simulink model "HANcoder_E407_TTA_Group2"  (R2018b)
settings: Solver=FixedStepDiscrete  StartTime=0.0  StopTime=1  FixedStep=0.01  RelTol=1e-3
PreLoadFcn:
  | librarySetup
  | eval([bdroot,'_startup']) %Calling [modelName]_startup.m
values from neighbouring files (symbols this model uses):
  BackUp_Role = 4    [HANcoder_E407_TTA_Group2_startup.m]
  basic_cycle_duration_bc0 = TM_Reset_Board   + COMP_duration    (= 550)    [HANcoder_E407_TTA_Group2_startup.m]    (also in HANcoder_E407_TTA_Template_startup.m = 212)
  basic_cycle_duration_bc1 = TM_Reset_Var_bc1 + COMP_duration    (= 610)    [HANcoder_E407_TTA_Group2_startup.m]    (also in HANcoder_E407_TTA_Template_startup.m = 212)
  board1_online = Simulink.Parameter    [HANcoder_E407_TTA_Group2_startup.m]
  board2_online = Simulink.Parameter    [HANcoder_E407_TTA_Group2_startup.m]
  board3_online = Simulink.Parameter    [HANcoder_E407_TTA_Group2_startup.m]
  board4_online = Simulink.Parameter    [HANcoder_E407_TTA_Group2_startup.m]
  comm_delay_estimation1 = round(comm_delay_measured1*hardware_granularity/frequency_IRQ)    [HANcoder_E407_TTA_Group2_startup.m]    (also in HANcoder_E407_TTA_Template_startup.m)
  comm_delay_estimation2 = round(comm_delay_measured2*hardware_granularity/frequency_IRQ)    [HANcoder_E407_TTA_Group2_startup.m]    (also in HANcoder_E407_TTA_Template_startup.m)
  COMM_Period = 50    [HANcoder_E407_TTA_Group2_startup.m]    (also in HANcoder_E407_TTA_Template_startup.m = 40)
  COMM_Phase1 = Simulink.Parameter    [HANcoder_E407_TTA_Group2_startup.m]    (also in HANcoder_E407_TTA_Template_startup.m)
  COMM_Phase2 = Simulink.Parameter    [HANcoder_E407_TTA_Group2_startup.m]    (also in HANcoder_E407_TTA_Template_startup.m)
  COMM_Phase_init1 = Simulink.Parameter    [HANcoder_E407_TTA_Group2_startup.m]    (also in HANcoder_E407_TTA_Template_startup.m)
  COMM_Phase_init2 = Simulink.Parameter    [HANcoder_E407_TTA_Group2_startup.m]    (also in HANcoder_E407_TTA_Template_startup.m)
  COMP_duration = 20    [HANcoder_E407_TTA_Group2_startup.m]    (also in HANcoder_E407_TTA_Template_startup.m = 4)
  Controller1_Board = 1    [HANcoder_E407_TTA_Group2_startup.m]    (also in HANcoder_E407_TTA_Template_startup.m)
  Controller2_Board = 2    [HANcoder_E407_TTA_Group2_startup.m]    (also in HANcoder_E407_TTA_Template_startup.m)
  Controller3_Board = 3    [HANcoder_E407_TTA_Group2_startup.m]    (also in HANcoder_E407_TTA_Template_startup.m)
  Controller4_Board = 4    [HANcoder_E407_TTA_Group2_startup.m]
  delta_a_set = Simulink.Parameter    [HANcoder_E407_TTA_Group2_startup.m]
  delta_f_set = Simulink.Parameter    [HANcoder_E407_TTA_Group2_startup.m]
  delta_max = 1    [HANcoder_E407_TTA_Group2_startup.m]
  delta_min = -1    [HANcoder_E407_TTA_Group2_startup.m]
  delta_precision = 6    [HANcoder_E407_TTA_Group2_startup.m]
  e_width = 0.1    [HANcoder_E407_TTA_Group2_startup.m]
  ErrorLog_ID = 31    [HANcoder_E407_TTA_Group2_startup.m]
  frequency_IRQ = 100    [HANcoder_E407_TTA_Group2_startup.m]    (also in HANcoder_E407_TTA_Template_startup.m)
  HANtuneOverride = Simulink.Parameter    [HANcoder_E407_TTA_Group2_startup.m]    (also in HANcoder_E407_TTA_Template_startup.m)
  hardware_granularity = 1000000    [HANcoder_E407_TTA_Group2_startup.m]    (also in HANcoder_E407_TTA_Template_startup.m)
  I_a = 2.25    [HANcoder_E407_TTA_Group2_startup.m]
  I_f = 2.25    [HANcoder_E407_TTA_Group2_startup.m]
  idle_time_init = basic_cycle_duration_bc0 + basic_cycle_duration_bc1    (= 1160)    [HANcoder_E407_TTA_Group2_startup.m]    (also in HANcoder_E407_TTA_Template_startup.m = 424)
  Input_Gen_Board = 5    [HANcoder_E407_TTA_Group2_startup.m]
  LA_Clock_Gr = 1    [HANcoder_E407_TTA_Group2_startup.m]    (also in HANcoder_E407_TTA_Template_startup.m)
  LA_COMM_dly = 1    [HANcoder_E407_TTA_Group2_startup.m]    (also in HANcoder_E407_TTA_Template_startup.m)
  LA_COMM_Err = 1    [HANcoder_E407_TTA_Group2_startup.m]    (also in HANcoder_E407_TTA_Template_startup.m)
  LA_E_Desync = 1    [HANcoder_E407_TTA_Group2_startup.m]    (also in HANcoder_E407_TTA_Template_startup.m)
  LA_MEX_Flag = 1    [HANcoder_E407_TTA_Group2_startup.m]    (also in HANcoder_E407_TTA_Template_startup.m)
  LA_Task_Act = 1    [HANcoder_E407_TTA_Group2_startup.m]    (also in HANcoder_E407_TTA_Template_startup.m)
  m_v = 100.0    (= 100)    [HANcoder_E407_TTA_Group2_startup.m]
  Master_Role = 1    [HANcoder_E407_TTA_Group2_startup.m]    (also in HANcoder_E407_TTA_Template_startup.m)
  matrix_cycle_duration = basic_cycle_duration_bc0 + basic_cycle_duration_bc1    (= 1160)    [HANcoder_E407_TTA_Group2_startup.m]    (also in HANcoder_E407_TTA_Template_startup.m = 424)
  matrix_rows = 2    [HANcoder_E407_TTA_Group2_startup.m]    (also in HANcoder_E407_TTA_Template_startup.m)
  max_desync = 15    [HANcoder_E407_TTA_Group2_startup.m]    (also in HANcoder_E407_TTA_Template_startup.m)
  max_num_msgs_CAN1 = 2^Tx_bit_number-1    (= 7)    [HANcoder_E407_TTA_Group2_startup.m]    (also in HANcoder_E407_TTA_Template_startup.m)
  max_num_msgs_CAN2 = max_num_msgs_CAN1    (= 7)    [HANcoder_E407_TTA_Group2_startup.m]    (also in HANcoder_E407_TTA_Template_startup.m)
  min_desync = (-1)*max_desync    (= -15)    [HANcoder_E407_TTA_Group2_startup.m]    (also in HANcoder_E407_TTA_Template_startup.m)
  OutControl1_ID = 23    [HANcoder_E407_TTA_Group2_startup.m]    (also in HANcoder_E407_TTA_Template_startup.m)
  OutControl2_ID = 24    [HANcoder_E407_TTA_Group2_startup.m]    (also in HANcoder_E407_TTA_Template_startup.m)
  OutEmulator_ID = 25    [HANcoder_E407_TTA_Group2_startup.m]    (also in HANcoder_E407_TTA_Template_startup.m)
  R_al = 0.10    (= 0.1)    [HANcoder_E407_TTA_Group2_startup.m]
  R_ar = 0.10    (= 0.1)    [HANcoder_E407_TTA_Group2_startup.m]
  R_fl = 0.10    (= 0.1)    [HANcoder_E407_TTA_Group2_startup.m]
  R_fr = 0.10    (= 0.1)    [HANcoder_E407_TTA_Group2_startup.m]
  script_run = Simulink.Parameter    [HANcoder_E407_TTA_Group2_startup.m]    (also in HANcoder_E407_TTA_Template_startup.m)
  SensorValues_ID = 22    [HANcoder_E407_TTA_Group2_startup.m]    (also in HANcoder_E407_TTA_Template_startup.m)
  SetValues_ID = 21    [HANcoder_E407_TTA_Group2_startup.m]    (also in HANcoder_E407_TTA_Template_startup.m)
  Slave_Role = 3    [HANcoder_E407_TTA_Group2_startup.m]    (also in HANcoder_E407_TTA_Template_startup.m = 2)
  speed_k_d = Simulink.Parameter    [HANcoder_E407_TTA_Group2_startup.m]
  speed_k_i = Simulink.Parameter    [HANcoder_E407_TTA_Group2_startup.m]
  speed_k_p = Simulink.Parameter    [HANcoder_E407_TTA_Group2_startup.m]
  speed_max = 10    [HANcoder_E407_TTA_Group2_startup.m]
  speed_min = -10    [HANcoder_E407_TTA_Group2_startup.m]
  speed_precision = 3    [HANcoder_E407_TTA_Group2_startup.m]
  Sync_ID = 1    [HANcoder_E407_TTA_Group2_startup.m]    (also in HANcoder_E407_TTA_Template_startup.m)
  tau_max = 5    [HANcoder_E407_TTA_Group2_startup.m]
  tau_min = -5    [HANcoder_E407_TTA_Group2_startup.m]
  tau_range = abs(tau_max) + abs(tau_min)    [HANcoder_E407_TTA_Group2_startup.m]
  theta_max = (speed_max/R_fr)*matrix_cycle_duration*frequency_IRQ/hardware_granularity    (= 11.6)    [HANcoder_E407_TTA_Group2_startup.m]
  theta_min = (-1)*theta_max    (= -11.6)    [HANcoder_E407_TTA_Group2_startup.m]
  theta_precision = 7-(fix(log2(theta_max))+1)    [HANcoder_E407_TTA_Group2_startup.m]
  Tl_a = 0.6    [HANcoder_E407_TTA_Group2_startup.m]
  Tl_f = 0.6    [HANcoder_E407_TTA_Group2_startup.m]
  TM_bc0_1 = basic_cycle_start    (= 0)    [HANcoder_E407_TTA_Group2_startup.m]
  TM_bc0_10 = TM_bc0_9 + COMP_duration    (= 270)    [HANcoder_E407_TTA_Group2_startup.m]
  TM_bc0_11 = TM_bc0_10 + COMP_duration    (= 290)    [HANcoder_E407_TTA_Group2_startup.m]
  TM_bc0_12 = TM_bc0_11  + COMM_duration    (= 340)    [HANcoder_E407_TTA_Group2_startup.m]
  TM_bc0_13 = TM_bc0_12 + COMP_duration    (= 360)    [HANcoder_E407_TTA_Group2_startup.m]
  TM_bc0_14 = TM_bc0_13 + COMP_duration    (= 380)    [HANcoder_E407_TTA_Group2_startup.m]
  TM_bc0_15 = TM_bc0_14  + COMM_duration    (= 430)    [HANcoder_E407_TTA_Group2_startup.m]
  TM_bc0_16 = TM_bc0_15 + COMP_duration    (= 450)    [HANcoder_E407_TTA_Group2_startup.m]
  TM_bc0_17 = TM_bc0_16 + COMP_duration    (= 470)    [HANcoder_E407_TTA_Group2_startup.m]
  TM_bc0_18 = TM_bc0_17 + COMP_duration    (= 490)    [HANcoder_E407_TTA_Group2_startup.m]
  TM_bc0_2 = TM_bc0_1   + COMM_duration    (= 50)    [HANcoder_E407_TTA_Group2_startup.m]
  TM_bc0_3 = TM_bc0_2  + COMP_duration    (= 70)    [HANcoder_E407_TTA_Group2_startup.m]
  TM_bc0_3_2 = TM_bc0_3   + 2    (= 72)    [HANcoder_E407_TTA_Group2_startup.m]
  TM_bc0_4 = TM_bc0_3   + COMP_duration    (= 90)    [HANcoder_E407_TTA_Group2_startup.m]
  TM_bc0_4_2 = TM_bc0_4    + 2    (= 92)    [HANcoder_E407_TTA_Group2_startup.m]
  TM_bc0_5 = TM_bc0_4    + COMP_duration    (= 110)    [HANcoder_E407_TTA_Group2_startup.m]
  TM_bc0_6 = TM_bc0_5  + COMM_duration    (= 160)    [HANcoder_E407_TTA_Group2_startup.m]
  TM_bc0_7 = TM_bc0_6 + COMP_duration    (= 180)    [HANcoder_E407_TTA_Group2_startup.m]
  TM_bc0_8 = TM_bc0_7 + COMP_duration    (= 200)    [HANcoder_E407_TTA_Group2_startup.m]
  TM_bc0_9 = TM_bc0_8  + COMM_duration    (= 250)    [HANcoder_E407_TTA_Group2_startup.m]
  TM_bc0_9_2 = TM_bc0_9 + 2    (= 252)    [HANcoder_E407_TTA_Group2_startup.m]
  TM_bc1_18 = TM_Check_Output_Emulator + COMP_duration    (= 520)    [HANcoder_E407_TTA_Group2_startup.m]
  TM_bc1_19 = TM_bc1_18 + COMM_duration    (= 570)    [HANcoder_E407_TTA_Group2_startup.m]
  TM_bc1_19_2 = TM_bc1_19 + 2    (= 572)    [HANcoder_E407_TTA_Group2_startup.m]
  TM_Check_Output_Control1 = TM_COMM_Output_Control1 + COMP_duration    (= 340)    [HANcoder_E407_TTA_Group2_startup.m]
  TM_Check_Output_Control2 = TM_COMM_Output_Control2 + COMM_duration    (= 410)    [HANcoder_E407_TTA_Group2_startup.m]
  TM_Check_Output_Emulator = TM_COMM_Output_Emulator + COMM_duration    (= 500)    [HANcoder_E407_TTA_Group2_startup.m]
  TM_Check_Output_Emulator_2 = TM_Check_Output_Emulator + 2    (= 502)    [HANcoder_E407_TTA_Group2_startup.m]
  TM_Check_Sensor_Values = TM_COMM_Sensor_Values + COMM_duration    (= 210)    [HANcoder_E407_TTA_Group2_startup.m]
  TM_Check_Sensor_Values_2 = TM_Check_Sensor_Values + 2    (= 212)    [HANcoder_E407_TTA_Group2_startup.m]
  TM_Check_Set_Values = TM_COMM_Set_Values + COMM_duration    (= 140)    [HANcoder_E407_TTA_Group2_startup.m]
  TM_Check_Set_Values_2 = TM_Check_Set_Values + 2    (= 142)    [HANcoder_E407_TTA_Group2_startup.m]
  TM_COMM_Output_Control1 = TM_Velocity + COMM_duration    (= 320)    [HANcoder_E407_TTA_Group2_startup.m]
  TM_COMM_Output_Control2 = TM_Check_Output_Control1 + COMP_duration    (= 360)    [HANcoder_E407_TTA_Group2_startup.m]
  TM_COMM_Output_Emulator = TM_TMR + COMP_duration    (= 450)    [HANcoder_E407_TTA_Group2_startup.m]
  TM_COMM_Sensor_Values = TM_Check_Set_Values + COMP_duration    (= 160)    [HANcoder_E407_TTA_Group2_startup.m]
  TM_COMM_Set_Values = TM_bc0_3 + COMP_duration    (= 90)    [HANcoder_E407_TTA_Group2_startup.m]
  TM_COMM_Sync = basic_cycle_start    (= 0)    [HANcoder_E407_TTA_Group2_startup.m]    (also in HANcoder_E407_TTA_Template_startup.m)
  TM_Data_bc0 = TM_COMM_Sync    (= 0)    [HANcoder_E407_TTA_Group2_startup.m]    (also in HANcoder_E407_TTA_Template_startup.m)
  TM_Data_bc1 = TM_Data_bc0(1:4)    [HANcoder_E407_TTA_Group2_startup.m]    (also in HANcoder_E407_TTA_Template_startup.m)
  TM_Reset_Board = TM_Reset_Var   + COMP_duration    (= 530)    [HANcoder_E407_TTA_Group2_startup.m]    (also in HANcoder_E407_TTA_Template_startup.m = 208)
  TM_Reset_Var = TM_bc0_18  + COMP_duration    (= 510)    [HANcoder_E407_TTA_Group2_startup.m]    (also in HANcoder_E407_TTA_Template_startup.m = 204)
  TM_Reset_Var_bc1 = TM_bc1_19 + COMP_duration    (= 590)    [HANcoder_E407_TTA_Group2_startup.m]    (also in HANcoder_E407_TTA_Template_startup.m = 200)
  TM_Reset_Var_bc1_2 = TM_Reset_Var_bc1 + 2    (= 592)    [HANcoder_E407_TTA_Group2_startup.m]    (also in HANcoder_E407_TTA_Template_startup.m = 202)
  TM_Steer = TM_Check_Sensor_Values + COMP_duration    (= 230)    [HANcoder_E407_TTA_Group2_startup.m]
  TM_TMR = TM_Check_Output_Control2 + COMP_duration    (= 430)    [HANcoder_E407_TTA_Group2_startup.m]
  TM_TMR_2 = TM_TMR + 1    (= 431)    [HANcoder_E407_TTA_Group2_startup.m]
  ... (+19 more)
undefined symbols (not defined in the file or in its folder): A0, A1, A2, A3, A4, CON2, CON4, D10, D12, D13, D8, D9
libraries: hdlsllib x340, HANcoder_STM32_Target x28, simulink x5, simulink_extras x1
(part 21 of 36)

== system HANcoder_E407_TTA_Group2/HANcoder STM32 Target - E407-STM32 algorithm/TTA CAN System/TTA System/Matrix Cycle Manager/Controller Matrix Cycle/controller basic cycle 0/COMM Task - Vote4/Transmission subtasks/Check msg transmission CAN1 ==
  note: The TX buffers are updated one tick
      | before the message is sent
  note: A message should be sent during
      | this tick through CAN1
  note: In the next tick, a message will be
      | sent through CAN1
  Local Time : Inport
  Time Mark : Inport  Port=2
  Tx_ID : Inport  Port=3
  Value Domain Msg : Inport  Port=4
  Enable : EnablePort
  Constant : Constant  Value=COMM_Phase_init1
  Constant11 : Constant  Value=0
  Constant22 : Constant
  Constant24 : Constant  Value=COMM_Phase1
  Constant27 : Constant  Value=COMM_Phase1
  Constant8 : Constant  Value=0
  Equal4 : RelationalOperator  Operator===  OutDataTypeStr=boolean  RndMeth=Simplest
  Equal7 : RelationalOperator  Operator===  OutDataTypeStr=boolean  RndMeth=Simplest
  Minus : Sum  Inputs=++-
  Minus1 : Sum  Inputs=+-
  Minus2 : Sum
  Mod : Math  Operator=mod  SaturateOnIntegerOverflow=on
  Mod1 : Math  Operator=mod  SaturateOnIntegerOverflow=on
  TX buffer update CAN1 : Subsystem  Priority=20
  Send CAN1 : Outport  OutputWhenDisabled=reset  InitialOutput=0
  wires:
  Equal4/1 -> TX buffer update CAN1/Enable
  Constant22/1 -> Minus/2
  Local Time/1 -> Minus1/1, Minus/1
  Tx_ID/1 -> TX buffer update CAN1/1(Tx_ID)
  Mod1/1 -> Equal7/1
  Constant27/1 -> Mod1/2
  Minus/1 -> Mod/1
  Value Domain Msg/1 -> TX buffer update CAN1/2(Msg_Value_Data)
  Constant24/1 -> Mod/2
  Mod/1 -> Equal4/1
  Minus1/1 -> Mod1/1
  Constant11/1 -> Equal7/2
  Equal7/1 -> Send CAN1/1
  Constant8/1 -> Equal4/2
  Constant/1 -> Minus2/2
  Minus2/1 -> Minus1/2, Minus/3
  Time Mark/1 -> Minus2/1

== system HANcoder_E407_TTA_Group2/HANcoder STM32 Target - E407-STM32 algorithm/TTA CAN System/TTA System/Matrix Cycle Manager/Controller Matrix Cycle/controller basic cycle 0/COMM Task - Vote4/Transmission subtasks/Check msg transmission CAN2 ==
  note: In the next tick, a message will be
      | sent through CAN2
  note: A message should be sent during
      | this tick through CAN2
  note: The TX buffers are updated one tick
      | before the message is sent
  Local Time : Inport
  Time Mark : Inport  Port=2
  Tx_ID : Inport  Port=3
  Value Domain Msg : Inport  Port=4
  Enable : EnablePort
  Constant : Constant  Value=COMM_Phase_init2
  Constant11 : Constant  Value=0
  Constant22 : Constant
  Constant24 : Constant  Value=COMM_Phase2
  Constant27 : Constant  Value=COMM_Phase2
  Constant8 : Constant  Value=0
  Equal4 : RelationalOperator  Operator===  OutDataTypeStr=boolean  RndMeth=Simplest
  Equal7 : RelationalOperator  Operator===  OutDataTypeStr=boolean  RndMeth=Simplest
  Minus : Sum  Inputs=++-
  Minus1 : Sum  Inputs=+-
  Minus2 : Sum
  Mod : Math  Operator=mod  SaturateOnIntegerOverflow=on
  Mod1 : Math  Operator=mod  SaturateOnIntegerOverflow=on
  TX buffer update CAN2 : Subsystem  Priority=20
  Send CAN2 : Outport  OutputWhenDisabled=reset  InitialOutput=0
  wires:
  Constant8/1 -> Equal4/2
  Equal7/1 -> Send CAN2/1
  Constant11/1 -> Equal7/2
  Minus1/1 -> Mod1/1
  Mod/1 -> Equal4/1
  Constant24/1 -> Mod/2
  Value Domain Msg/1 -> TX buffer update CAN2/2(Msg_Value_Data)
  Minus/1 -> Mod/1
  Constant27/1 -> Mod1/2
  Mod1/1 -> Equal7/1
  Tx_ID/1 -> TX buffer update CAN2/1(Tx_ID)
  Local Time/1 -> Minus/1, Minus1/1
  Constant22/1 -> Minus/2
  Equal4/1 -> TX buffer update CAN2/Enable
  Constant/1 -> Minus2/2
  Time Mark/1 -> Minus2/1
  Minus2/1 -> Minus1/2, Minus/3

== system HANcoder_E407_TTA_Group2/HANcoder STM32 Target - E407-STM32 algorithm/TTA CAN System/TTA System/Matrix Cycle Manager/Controller Matrix Cycle/controller basic cycle 0/COMM Task - Vote4/Transmission subtasks/Msg_Value_Data_Encoded ==
  note: Value domain message encoding
      | <Warning!> The first buffer (from the top) is not used in transmission!
  Enable : EnablePort
  Bus Creator : BusCreator  Inputs=8  OutDataTypeStr=Bus: msg_buffer_type
  Constant : Constant  Value=0  OutDataTypeStr=uint8
  Data Store Read : DataStoreRead  DataStoreName=Own_Vote
  Value_domain_msg : Outport
  wires:
  Bus Creator/1 -> Value_domain_msg/1
  Constant/1 -> Bus Creator/3, Bus Creator/4, Bus Creator/5, Bus Creator/6, Bus Creator/7, Bus Creator/8, Bus Creator/1
  Data Store Read/1 -> Bus Creator/2

== system HANcoder_E407_TTA_Group2/HANcoder STM32 Target - E407-STM32 algorithm/TTA CAN System/TTA System/Matrix Cycle Manager/Controller Matrix Cycle/controller basic cycle 0/COMP Task - Check Timeouts/Timeout and Board error counter/Timeout Counter 1 DEBUG ==
  Timeout : Inport
  Constant : Constant
  Data Store Memory : DataStoreMemory  DataStoreName=BC0_TM1_timeout_counter  ReadBeforeWriteMsg=warning  WriteAfterWriteMsg=warning  WriteAfterReadMsg=warning  ShowAdditionalParam=off
  Data Store Read : DataStoreRead  DataStoreName=BC0_TM1_timeout_counter
  Data Store Read1 : DataStoreRead  DataStoreName=BC0_TM1_timeout_counter
  Data Store Write : DataStoreWrite  DataStoreName=BC0_TM1_timeout_counter
  Plus : Sum
  Switch : Switch  Criteria=u2 > Threshold
  wires:
  Timeout/1 -> Switch/2
  Switch/1 -> Data Store Write/1  "TM1_timeout_counter_s"
  Data Store Read1/1 -> Plus/1
  Constant/1 -> Plus/2
  Plus/1 -> Switch/1
  Data Store Read/1 -> Switch/3

== system HANcoder_E407_TTA_Group2/HANcoder STM32 Target - E407-STM32 algorithm/TTA CAN System/TTA System/Matrix Cycle Manager/Controller Matrix Cycle/controller basic cycle 0/COMP Task - Check Timeouts/Timeout and Board error counter/Timeout Counter 2 DEBUG ==
  Timeout : Inport
  Constant : Constant
  Data Store Memory : DataStoreMemory  DataStoreName=BC0_TM2_timeout_counter  ReadBeforeWriteMsg=warning  WriteAfterWriteMsg=warning  WriteAfterReadMsg=warning  ShowAdditionalParam=off
  Data Store Read : DataStoreRead  DataStoreName=BC0_TM2_timeout_counter
  Data Store Read1 : DataStoreRead  DataStoreName=BC0_TM2_timeout_counter
  Data Store Write : DataStoreWrite  DataStoreName=BC0_TM2_timeout_counter
  Plus : Sum
  Switch : Switch  Criteria=u2 > Threshold
  wires:
  Data Store Read/1 -> Switch/3
  Plus/1 -> Switch/1
  Constant/1 -> Plus/2
  Data Store Read1/1 -> Plus/1
  Switch/1 -> Data Store Write/1  "TM2_timeout_counter_s"
  Timeout/1 -> Switch/2

== system HANcoder_E407_TTA_Group2/HANcoder STM32 Target - E407-STM32 algorithm/TTA CAN System/TTA System/Matrix Cycle Manager/Controller Matrix Cycle/controller basic cycle 0/COMP Task - Check Timeouts/Timeout and Board error counter/Timeout Counter 3 DEBUG ==
  Timeout : Inport
  Constant : Constant
  Data Store Memory : DataStoreMemory  DataStoreName=BC0_TM3_timeout_counter  ReadBeforeWriteMsg=warning  WriteAfterWriteMsg=warning  WriteAfterReadMsg=warning  ShowAdditionalParam=off
  Data Store Read : DataStoreRead  DataStoreName=BC0_TM3_timeout_counter
  Data Store Read1 : DataStoreRead  DataStoreName=BC0_TM3_timeout_counter
  Data Store Write : DataStoreWrite  DataStoreName=BC0_TM3_timeout_counter
  Plus : Sum
  Switch : Switch  Criteria=u2 > Threshold
  wires:
  Timeout/1 -> Switch/2
  Switch/1 -> Data Store Write/1  "TM3_timeout_counter_s"
  Data Store Read1/1 -> Plus/1
  Constant/1 -> Plus/2
  Plus/1 -> Switch/1
  Data Store Read/1 -> Switch/3

== system HANcoder_E407_TTA_Group2/HANcoder STM32 Target - E407-STM32 algorithm/TTA CAN System/TTA System/Matrix Cycle Manager/Controller Matrix Cycle/controller basic cycle 0/COMP Task - Check Timeouts/Timeout and Board error counter/Timeout Counter 4 DEBUG ==
  Timeout : Inport
  Constant : Constant
  Data Store Memory : DataStoreMemory  DataStoreName=BC0_TM4_timeout_counter  ReadBeforeWriteMsg=warning  WriteAfterWriteMsg=warning  WriteAfterReadMsg=warning  ShowAdditionalParam=off
  Data Store Read : DataStoreRead  DataStoreName=BC0_TM4_timeout_counter
  Data Store Read1 : DataStoreRead  DataStoreName=BC0_TM4_timeout_counter
  Data Store Write : DataStoreWrite  DataStoreName=BC0_TM4_timeout_counter
  Plus : Sum
  Switch : Switch  Criteria=u2 > Threshold
  wires:
  Timeout/1 -> Switch/2
  Switch/1 -> Data Store Write/1  "TM4_timeout_counter_s"
  Data Store Read1/1 -> Plus/1
  Constant/1 -> Plus/2
  Plus/1 -> Switch/1
  Data Store Read/1 -> Switch/3

== system HANcoder_E407_TTA_Group2/HANcoder STM32 Target - E407-STM32 algorithm/TTA CAN System/TTA System/Matrix Cycle Manager/Controller Matrix Cycle/controller basic cycle 0/COMP Task - New Master/New Master/Enabled Subsystem ==
  In1 : Inport
  Enable : EnablePort
  Out1 : Outport
  wires:
  In1/1 -> Out1/1

== system HANcoder_E407_TTA_Group2/HANcoder STM32 Target - E407-STM32 algorithm/TTA CAN System/TTA System/Matrix Cycle Manager/Controller Matrix Cycle/controller basic cycle 0/COMP Task - New Master/New Master/Votes recount to choose Master ==
  note: If no votes received: RESET Board
  note: Add self node vote
  Abs : Abs
  Compare To Constant : simulink/Logic and Bit Operations/Compare To Constant  relop===  const=0  OutDataTypeStr=boolean
  Compare To Constant1 : simulink/Logic and Bit Operations/Compare To Constant  relop=<  const=0  OutDataTypeStr=boolean
  Compare To Constant3 : simulink/Logic and Bit Operations/Compare To Constant  relop===  const=0  OutDataTypeStr=boolean
  Constant : Constant  Value=0
  Constant1 : Constant  Priority=8  Value=2
  Constant2 : Constant  Priority=8
  Constant3 : Constant  Priority=8  Value=3
  Constant4 : Constant  Priority=8  Value=4
  Data Store Read25 : DataStoreRead  DataStoreName=Votes_count  DataStoreElements=Votes_count.First_Board#Votes_count.Second_Board#Votes_count.Third_Board#Votes_count.Fourth_Board
  Data Store Read29 : DataStoreRead  DataStoreName=Own_Vote
  Equal{,1,17..19} (5 alike) : RelationalOperator  Operator===  OutDataTypeStr=boolean  RndMeth=Simplest
  Find Nonzero Elements : Find  NumberOfInputDimensions=3  IndexMode=Zero-based  OutDataTypeStr=int32
  Find Nonzero Elements1 : Find  NumberOfInputDimensions=3  IndexMode=Zero-based  OutDataTypeStr=int32
  Find Nonzero Elements2 : Find  NumberOfInputDimensions=3  IndexMode=Zero-based  OutDataTypeStr=int32
  Index Corrector : Constant
  Index Corrector1 : Constant
  Index Corrector2 : Constant
  Max : MinMax  Function=max
  Max1 : MinMax  Function=max
  Min : MinMax
  Min1 : MinMax
  Min3 : MinMax
  Min4 : MinMax  Function=max
  Minus : Sum
  Minus1 : Sum
  Minus2 : Sum
  Multiply : Product
  Mux : Mux
  Mux1 : Mux
  Plus{,1..3} (4 alike) : Sum
  Subtract : Sum  Inputs=+-
  Subtract1 : Sum  Inputs=+-
  Sum of Elements : Sum  Inputs=+
  Switch : Switch  Criteria=u2 > Threshold
  Master_ID : Outport
  "Voter_ID " : Outport  Port=2
  "BackUp_ID " : Outport  Port=3
  Reset Board : Outport  Port=4
  wires:
  Data Store Read25/1 -> Plus/1, Mux1/1
  Equal18/1 -> Plus1/2
  Plus/1 -> Mux/1  "Vote1_s"
  Plus1/1 -> Mux/2  "Vote2_s"
  Data Store Read25/2 -> Plus1/1, Mux1/2
  Plus2/1 -> Mux/3  "Vote3_s"
  Equal19/1 -> Plus2/2
  Equal17/1 -> Plus/2
  Max/1 -> Subtract/2
  Mux/1 -> Subtract/1, Max/1
  Data Store Read25/3 -> Plus2/1, Mux1/3
  Mux1/1 -> Max1/1
  Max1/1 -> Equal/2
  Constant/1 -> Equal/1
  Equal/1 -> Reset Board/1
  Data Store Read25/4 -> Plus3/1, Mux1/4
  Equal1/1 -> Plus3/2
  Data Store Read29/1 -> Equal1/2, Equal19/2, Equal18/2, Equal17/2
  Plus3/1 -> Mux/4  "Vote4_s"
  Constant2/1 -> Equal17/1
  Constant1/1 -> Equal18/1
  Constant3/1 -> Equal19/1
  Constant4/1 -> Equal1/1
  Subtract/1 -> Multiply/1, Subtract1/1, Min3/1, Compare To Constant/1
  Index Corrector2/1 -> Minus2/2
  Index Corrector/1 -> Minus/2
  Compare To Constant/1 -> Find Nonzero Elements/1
  Min/1 -> Minus/1
  Minus2/1 -> "BackUp_ID "/1
  Minus/1 -> Master_ID/1
  Find Nonzero Elements1/1 -> Switch/1
  Min1/1 -> Minus1/1
  Switch/1 -> Min1/1
  Find Nonzero Elements/1 -> Min/1
  Abs/1 -> Switch/2
  Minus1/1 -> "Voter_ID "/1
  Compare To Constant1/1 -> Find Nonzero Elements1/1
  Index Corrector1/1 -> Minus1/2
  Multiply/1 -> Compare To Constant1/1, Sum of Elements/1
  Min3/1 -> Subtract1/2
  Compare To Constant3/1 -> Find Nonzero Elements2/1
  Find Nonzero Elements2/1 -> Min4/1, Switch/3
  Subtract1/1 -> Compare To Constant3/1, Multiply/2
  Sum of Elements/1 -> Abs/1
  Min4/1 -> Minus2/1

== system HANcoder_E407_TTA_Group2/HANcoder STM32 Target - E407-STM32 algorithm/TTA CAN System/TTA System/Matrix Cycle Manager/Controller Matrix Cycle/controller basic cycle 0/COMP Task - Sync bc0 check/Process_Messages/Demux message CAN1 and check coherence ==
  CAN1_Rx_msg : Inport  OutDataTypeStr=Bus: msg_buffer_type
  expected_basic_cycle : Inport  Port=2
  expected_board_id : Inport  Port=3
  Enable : EnablePort
  AND : Logic  IconShape=distinctive  AllPortsSameDT=off  OutDataTypeStr=boolean
  Bus Creator : BusCreator  Inputs=8  OutDataTypeStr=Bus: msg_buffer_type
  Bus Selector : BusSelector  OutputSignals=Buffer_1,Buffer_2,Buffer_3,Buffer_4,Buffer_5,Buffer_6,Buffer_7,Buffer_8
  Constant : Constant  Value=0  OutDataTypeStr=uint8
  Equal : RelationalOperator  Operator===  OutDataTypeStr=boolean  RndMeth=Simplest
  Equal1 : RelationalOperator  Operator===  OutDataTypeStr=boolean  RndMeth=Simplest
  Subsystem : Subsystem
  msg_count>2_DEBUG : Subsystem
  CAN1_msg : Outport  OutDataTypeStr=Bus: msg_buffer_type
  Msg_Count_CAN1 : Outport  Port=2
  CAN1_msg_coherent : Outport  Port=3  OutputWhenDisabled=reset  InitialOutput=0
  wires:
  Bus Selector/2 -> Bus Creator/2  "<Buffer_2>"
  Bus Selector/3 -> Bus Creator/3  "<Buffer_3>"
  CAN1_Rx_msg/1 -> Bus Selector/1
  Equal/1 -> AND/2
  Equal1/1 -> AND/1
  AND/1 -> CAN1_msg_coherent/1
  expected_basic_cycle/1 -> Equal1/2
  expected_board_id/1 -> Equal/2
  Bus Selector/6 -> Bus Creator/6  "<Buffer_6>"
  Bus Selector/5 -> Bus Creator/5  "<Buffer_5>"
  Bus Selector/7 -> Bus Creator/7  "<Buffer_7>"
  Bus Selector/8 -> Bus Creator/8  "<Buffer_8>"
  Bus Selector/4 -> Bus Creator/4  "<Buffer_4>"
  Subsystem/3(board_id) -> Equal/1
  Bus Selector/1 -> Subsystem/1(Msg_Temporal_Data)  "<Buffer_1>"
  Subsystem/1(basic_cycle) -> Equal1/1
  Subsystem/2(msg_count) -> msg_count>2_DEBUG/1(msg_c), Msg_Count_CAN1/1
  Bus Creator/1 -> CAN1_msg/1
  Constant/1 -> Bus Creator/1

== system HANcoder_E407_TTA_Group2/HANcoder STM32 Target - E407-STM32 algorithm/TTA CAN System/TTA System/Matrix Cycle Manager/Controller Matrix Cycle/controller basic cycle 0/COMP Task - Sync bc0 check/Process_Messages/Demux message CAN1 and check coherence1 ==
  CAN2_Rx_msg : Inport  OutDataTypeStr=Bus: msg_buffer_type
  expected_basic_cycle : Inport  Port=2
  expected_board_id : Inport  Port=3
  Enable : EnablePort
  AND : Logic  IconShape=distinctive  AllPortsSameDT=off  OutDataTypeStr=boolean
  Bus Creator : BusCreator  Inputs=8  OutDataTypeStr=Bus: msg_buffer_type
  Bus Selector : BusSelector  OutputSignals=Buffer_1,Buffer_2,Buffer_3,Buffer_4,Buffer_5,Buffer_6,Buffer_7,Buffer_8
  Constant : Constant  Value=0  OutDataTypeStr=uint8
  Equal : RelationalOperator  Operator===  OutDataTypeStr=boolean  RndMeth=Simplest
  Equal1 : RelationalOperator  Operator===  OutDataTypeStr=boolean  RndMeth=Simplest
  Subsystem : Subsystem
  msg_count>2_DEBUG : Subsystem
  CAN2_msg_coherent : Outport  OutputWhenDisabled=reset  InitialOutput=0
  Msg_Count_CAN2 : Outport  Port=2
  CAN2_msg : Outport  Port=3  OutDataTypeStr=Bus: msg_buffer_type
  wires:
  Bus Selector/2 -> Bus Creator/2  "<Buffer_2>"
  Bus Selector/3 -> Bus Creator/3  "<Buffer_3>"
  CAN2_Rx_msg/1 -> Bus Selector/1
  Equal/1 -> AND/2
  Equal1/1 -> AND/1
  AND/1 -> CAN2_msg_coherent/1
  expected_basic_cycle/1 -> Equal1/2
  expected_board_id/1 -> Equal/2
  Bus Selector/6 -> Bus Creator/6  "<Buffer_6>"
  Bus Selector/5 -> Bus Creator/5  "<Buffer_5>"
  Bus Selector/7 -> Bus Creator/7  "<Buffer_7>"
  Bus Selector/8 -> Bus Creator/8  "<Buffer_8>"
  Bus Selector/4 -> Bus Creator/4  "<Buffer_4>"
  Subsystem/3(board_id) -> Equal/1
  Bus Selector/1 -> Subsystem/1(Msg_Temporal_Data)  "<Buffer_1>"
  Subsystem/1(basic_cycle) -> Equal1/1
  Subsystem/2(msg_count) -> msg_count>2_DEBUG/1(msg_c), Msg_Count_CAN2/1
  Bus Creator/1 -> CAN2_msg/1
  Constant/1 -> Bus Creator/1

== system HANcoder_E407_TTA_Group2/HANcoder STM32 Target - E407-STM32 algorithm/TTA CAN System/TTA System/Matrix Cycle Manager/Controller Matrix Cycle/controller basic cycle 0/COMP Task - Sync bc0 check/Process_Messages/Desync calculation ==
  note: Estimation of the Local Time when the message was sent
  note: Desync CAN2
      | expected RX - Actual RX
  note: Desync CAN1
      | expected RX - Actual RX
  TM_COMM : Inport
  New_msg_CAN1 : Inport  Port=2
  msg_count_CAN1 : Inport  Port=3
  msg_count_CAN2 : Inport  Port=4
  Enable : EnablePort
  Constant : Constant  Value=COMM_Phase1
  Constant1 : Constant  Value=COMM_Phase2
  Data Store Read : DataStoreRead  DataStoreName=Msg_Rx_Ticks_CAN1
  Data Store Read1 : DataStoreRead  DataStoreName=Msg_Rx_Ticks_CAN2
  Data Store Write1 : DataStoreWrite  Priority=23  DataStoreName=Desync_Ticks
  Minus : Sum  Priority=21  Inputs=+-
  Minus1 : Sum  Priority=20  Inputs=+-
  Multiply : Product  Priority=10
  Multiply1 : Product  Priority=12
  Saturation : Saturate  UpperLimit=max_desync  LowerLimit=min_desync
  Sum : Sum  Priority=11  Inputs=+++
  Sum1 : Sum  Priority=13  Inputs=+++
  Switch1 : Switch  Priority=22  Criteria=u2 > Threshold
  delay_estimation_1 : Constant  Value=comm_delay_estimation1
  delay_estimation_2 : Constant  Value=comm_delay_estimation2
  wires:
  TM_COMM/1 -> Sum1/2, Sum/2
  delay_estimation_1/1 -> Sum/3
  msg_count_CAN1/1 -> Multiply/2
  Switch1/1 -> Saturation/1
  Minus/1 -> Switch1/3
  Sum1/1 -> [expected_LT_CAN2]
  delay_estimation_2/1 -> Sum1/3
  Multiply1/1 -> Sum1/1
  [expected_LT_CAN1] -> Minus1/1
  [expected_LT_CAN2] -> Minus/1
  Data Store Read1/1 -> Minus/2
  Multiply/1 -> Sum/1
  Data Store Read/1 -> Minus1/2
  msg_count_CAN2/1 -> Multiply1/2
  Sum/1 -> [expected_LT_CAN1]
  Minus1/1 -> Switch1/1
  Constant/1 -> Multiply/1
  Constant1/1 -> Multiply1/1
  New_msg_CAN1/1 -> Switch1/2
  Saturation/1 -> Data Store Write1/1  "Desync_Sync_bc0_s"

== system HANcoder_E407_TTA_Group2/HANcoder STM32 Target - E407-STM32 algorithm/TTA CAN System/TTA System/Matrix Cycle Manager/Controller Matrix Cycle/controller basic cycle 0/COMP Task - Update LT/Local Time Update/Desync_Negative ==
  note: Local time correction when Desync is negative
      | In this case the Local Time "goes back in time".
      | Previous tasks will not be activated because
      | sync_processed flag is alread set.
  note: Current Local Time correction
  note: Local Time Update
  Current_Local_Time : Inport
  Enable : EnablePort
  Cast : DataTypeConversion  Priority=13  OutDataTypeStr=uint16
  Data Store Read : DataStoreRead  Priority=11  DataStoreName=Desync_Ticks
  Data Store Write1 : DataStoreWrite  Priority=14  DataStoreName=Local_Ticks  DataStoreElements=Local_Ticks
  Minus : Sum  Priority=12
  wires:
  Data Store Read/1 -> Minus/2
  Minus/1 -> Cast/1
  Cast/1 -> Data Store Write1/1
  Current_Local_Time/1 -> Minus/1

== system HANcoder_E407_TTA_Group2/HANcoder STM32 Target - E407-STM32 algorithm/TTA CAN System/TTA System/Matrix Cycle Manager/Controller Matrix Cycle/controller basic cycle 0/COMP Task - Vote Decision/Vote Decision/Ensure no self votes or failed master reelected ==
  Node ID : Inport
  Sync Timeout : Inport  Port=2
  Error counter : Inport  Port=3
  AND : Logic  IconShape=distinctive  AllPortsSameDT=off  OutDataTypeStr=boolean
  Data Store Read : DataStoreRead  DataStoreName=Board_ID
  Data Store Read2 : DataStoreRead  DataStoreName=Master_ID
  Equal1 : RelationalOperator  Operator===  OutDataTypeStr=boolean  RndMeth=Simplest
  Equal2 : RelationalOperator  Operator===  OutDataTypeStr=boolean  RndMeth=Simplest
  MAX error count : Constant  Value=4294967295  OutDataTypeStr=uint32
  NOT : Logic  Operator=NOT  IconShape=distinctive  AllPortsSameDT=off  OutDataTypeStr=boolean
  OR : Logic  Operator=OR  IconShape=distinctive  AllPortsSameDT=off  OutDataTypeStr=boolean
  Switch : Switch  Criteria=u2 > Threshold
  Out1 : Outport
  wires:
  Equal1/1 -> OR/1
  Data Store Read/1 -> Equal1/2
  MAX error count/1 -> Switch/1
  Switch/1 -> Out1/1
  Error counter/1 -> Switch/3
  Node ID/1 -> Equal1/1, Equal2/2
  Sync Timeout/1 -> NOT/1
  Data Store Read2/1 -> Equal2/1
  Equal2/1 -> AND/1
  NOT/1 -> AND/2
  AND/1 -> OR/2
  OR/1 -> Switch/2

== system HANcoder_E407_TTA_Group2/HANcoder STM32 Target - E407-STM32 algorithm/TTA CAN System/TTA System/Matrix Cycle Manager/Controller Matrix Cycle/controller basic cycle 0/COMP Task - Vote Decision/Vote Decision/Ensure no self votes or failed master reelected1 ==
  Node ID : Inport
  Sync Timeout : Inport  Port=2
  Error counter : Inport  Port=3
  AND : Logic  IconShape=distinctive  AllPortsSameDT=off  OutDataTypeStr=boolean
  Data Store Read : DataStoreRead  DataStoreName=Board_ID
  Data Store Read2 : DataStoreRead  DataStoreName=Master_ID
  Equal1 : RelationalOperator  Operator===  OutDataTypeStr=boolean  RndMeth=Simplest
  Equal2 : RelationalOperator  Operator===  OutDataTypeStr=boolean  RndMeth=Simplest
  MAX error count : Constant  Value=4294967295  OutDataTypeStr=uint32
  NOT : Logic  Operator=NOT  IconShape=distinctive  AllPortsSameDT=off  OutDataTypeStr=boolean
  OR : Logic  Operator=OR  IconShape=distinctive  AllPortsSameDT=off  OutDataTypeStr=boolean
  Switch : Switch  Criteria=u2 > Threshold
  Out1 : Outport
  wires:
  OR/1 -> Switch/2
  AND/1 -> OR/2
  NOT/1 -> AND/2
  Equal2/1 -> AND/1
  Data Store Read2/1 -> Equal2/1
  Sync Timeout/1 -> NOT/1
  Node ID/1 -> Equal2/2, Equal1/1
  Error counter/1 -> Switch/3
  Switch/1 -> Out1/1
  MAX error count/1 -> Switch/1
  Data Store Read/1 -> Equal1/2
  Equal1/1 -> OR/1

== system HANcoder_E407_TTA_Group2/HANcoder STM32 Target - E407-STM32 algorithm/TTA CAN System/TTA System/Matrix Cycle Manager/Controller Matrix Cycle/controller basic cycle 0/COMP Task - Vote Decision/Vote Decision/Ensure no self votes or failed master reelected2 ==
  Node ID : Inport
  Sync Timeout : Inport  Port=2
  Error counter : Inport  Port=3
  AND : Logic  IconShape=distinctive  AllPortsSameDT=off  OutDataTypeStr=boolean
  Data Store Read : DataStoreRead  DataStoreName=Board_ID
  Data Store Read2 : DataStoreRead  DataStoreName=Master_ID
  Equal1 : RelationalOperator  Operator===  OutDataTypeStr=boolean  RndMeth=Simplest
  Equal2 : RelationalOperator  Operator===  OutDataTypeStr=boolean  RndMeth=Simplest
  MAX error count : Constant  Value=4294967295  OutDataTypeStr=uint32
  NOT : Logic  Operator=NOT  IconShape=distinctive  AllPortsSameDT=off  OutDataTypeStr=boolean
  OR : Logic  Operator=OR  IconShape=distinctive  AllPortsSameDT=off  OutDataTypeStr=boolean
  Switch : Switch  Criteria=u2 > Threshold
  Out1 : Outport
  wires:
  Equal1/1 -> OR/1
  Data Store Read/1 -> Equal1/2
  MAX error count/1 -> Switch/1
  Switch/1 -> Out1/1
  Error counter/1 -> Switch/3
  Node ID/1 -> Equal1/1, Equal2/2
  Sync Timeout/1 -> NOT/1
  Data Store Read2/1 -> Equal2/1
  Equal2/1 -> AND/1
  NOT/1 -> AND/2
  AND/1 -> OR/2
  OR/1 -> Switch/2

== system HANcoder_E407_TTA_Group2/HANcoder STM32 Target - E407-STM32 algorithm/TTA CAN System/TTA System/Matrix Cycle Manager/Controller Matrix Cycle/controller basic cycle 0/COMP Task - Vote Decision/Vote Decision/Ensure no self votes or failed master reelected3 ==
  Node ID : Inport
  Sync Timeout : Inport  Port=2
  Error counter : Inport  Port=3
  AND : Logic  IconShape=distinctive  AllPortsSameDT=off  OutDataTypeStr=boolean
  Data Store Read : DataStoreRead  DataStoreName=Board_ID
  Data Store Read2 : DataStoreRead  DataStoreName=Master_ID
  Equal1 : RelationalOperator  Operator===  OutDataTypeStr=boolean  RndMeth=Simplest
  Equal2 : RelationalOperator  Operator===  OutDataTypeStr=boolean  RndMeth=Simplest
  MAX error count : Constant  Value=4294967295  OutDataTypeStr=uint32
  NOT : Logic  Operator=NOT  IconShape=distinctive  AllPortsSameDT=off  OutDataTypeStr=boolean
  OR : Logic  Operator=OR  IconShape=distinctive  AllPortsSameDT=off  OutDataTypeStr=boolean
  Switch : Switch  Criteria=u2 > Threshold
  Out1 : Outport
  wires:
  Equal1/1 -> OR/1
  Data Store Read/1 -> Equal1/2
  MAX error count/1 -> Switch/1
  Switch/1 -> Out1/1
  Error counter/1 -> Switch/3
  Node ID/1 -> Equal1/1, Equal2/2
  Sync Timeout/1 -> NOT/1
  Data Store Read2/1 -> Equal2/1
  Equal2/1 -> AND/1
  NOT/1 -> AND/2
  AND/1 -> OR/2
  OR/1 -> Switch/2

== system HANcoder_E407_TTA_Group2/HANcoder STM32 Target - E407-STM32 algorithm/TTA CAN System/TTA System/Matrix Cycle Manager/Controller Matrix Cycle/controller basic cycle 0/COMP Task - Vote1 check/Process_Messages1/Demux message CAN1 and check coherence ==
  CAN1_Rx_msg : Inport  OutDataTypeStr=Bus: msg_buffer_type
  expected_board_id : Inport  Port=2
  Enable : EnablePort
  Bus Creator : BusCreator  Inputs=8  OutDataTypeStr=Bus: msg_buffer_type
  Bus Selector : BusSelector  OutputSignals=Buffer_1,Buffer_2,Buffer_3,Buffer_4,Buffer_5,Buffer_6,Buffer_7,Buffer_8
  Constant : Constant  Value=0  OutDataTypeStr=uint8
  Equal : RelationalOperator  Operator===  OutDataTypeStr=boolean  RndMeth=Simplest
  Subsystem : Subsystem
  Terminator : Terminator
  msg_count>2_DEBUG : Subsystem
  CAN1_msg : Outport  OutDataTypeStr=Bus: msg_buffer_type
  Msg_Count_CAN1 : Outport  Port=2
  CAN1_msg_coherent : Outport  Port=3  OutputWhenDisabled=reset  InitialOutput=0
  wires:
  Bus Selector/2 -> Bus Creator/2  "<Buffer_2>"
  Bus Selector/3 -> Bus Creator/3  "<Buffer_3>"
  CAN1_Rx_msg/1 -> Bus Selector/1
  Equal/1 -> CAN1_msg_coherent/1
  expected_board_id/1 -> Equal/2
  Bus Selector/6 -> Bus Creator/6  "<Buffer_6>"
  Bus Selector/5 -> Bus Creator/5  "<Buffer_5>"
  Bus Selector/7 -> Bus Creator/7  "<Buffer_7>"
  Bus Selector/8 -> Bus Creator/8  "<Buffer_8>"
  Bus Selector/4 -> Bus Creator/4  "<Buffer_4>"
  Subsystem/3(board_id) -> Equal/1
  Bus Selector/1 -> Subsystem/1(Msg_Temporal_Data)  "<Buffer_1>"
  Subsystem/2(msg_count) -> msg_count>2_DEBUG/1(msg_c), Msg_Count_CAN1/1
  Bus Creator/1 -> CAN1_msg/1
  Constant/1 -> Bus Creator/1
  Subsystem/1(basic_cycle) -> Terminator/1

== system HANcoder_E407_TTA_Group2/HANcoder STM32 Target - E407-STM32 algorithm/TTA CAN System/TTA System/Matrix Cycle Manager/Controller Matrix Cycle/controller basic cycle 0/COMP Task - Vote1 check/Process_Messages1/Demux message CAN1 and check coherence1 ==
  CAN2_Rx_msg : Inport  OutDataTypeStr=Bus: msg_buffer_type
  expected_board_id : Inport  Port=2
  Enable : EnablePort
  Bus Creator : BusCreator  Inputs=8  OutDataTypeStr=Bus: msg_buffer_type
  Bus Selector : BusSelector  OutputSignals=Buffer_1,Buffer_2,Buffer_3,Buffer_4,Buffer_5,Buffer_6,Buffer_7,Buffer_8
  Constant : Constant  Value=0  OutDataTypeStr=uint8
  Equal : RelationalOperator  Operator===  OutDataTypeStr=boolean  RndMeth=Simplest
  Subsystem : Subsystem
  Terminator : Terminator
  msg_count>2_DEBUG : Subsystem
  CAN2_msg_coherent : Outport  OutputWhenDisabled=reset  InitialOutput=0
  Msg_Count_CAN2 : Outport  Port=2
  CAN2_msg : Outport  Port=3  OutDataTypeStr=Bus: msg_buffer_type
  wires:
  Bus Selector/2 -> Bus Creator/2  "<Buffer_2>"
  Bus Selector/3 -> Bus Creator/3  "<Buffer_3>"
  CAN2_Rx_msg/1 -> Bus Selector/1
  Equal/1 -> CAN2_msg_coherent/1
  expected_board_id/1 -> Equal/2
  Bus Selector/6 -> Bus Creator/6  "<Buffer_6>"
  Bus Selector/5 -> Bus Creator/5  "<Buffer_5>"
  Bus Selector/7 -> Bus Creator/7  "<Buffer_7>"
  Bus Selector/8 -> Bus Creator/8  "<Buffer_8>"
  Bus Selector/4 -> Bus Creator/4  "<Buffer_4>"
  Subsystem/3(board_id) -> Equal/1
  Bus Selector/1 -> Subsystem/1(Msg_Temporal_Data)  "<Buffer_1>"
  Subsystem/2(msg_count) -> msg_count>2_DEBUG/1(msg_c), Msg_Count_CAN2/1
  Bus Creator/1 -> CAN2_msg/1
  Constant/1 -> Bus Creator/1
  Subsystem/1(basic_cycle) -> Terminator/1

== system HANcoder_E407_TTA_Group2/HANcoder STM32 Target - E407-STM32 algorithm/TTA CAN System/TTA System/Matrix Cycle Manager/Controller Matrix Cycle/controller basic cycle 0/COMP Task - Vote2 check/Process_Messages/Demux message CAN1 and check coherence ==
  CAN1_Rx_msg : Inport  OutDataTypeStr=Bus: msg_buffer_type
  expected_board_id : Inport  Port=2
  Enable : EnablePort
  Bus Creator : BusCreator  Inputs=8  OutDataTypeStr=Bus: msg_buffer_type
  Bus Selector : BusSelector  OutputSignals=Buffer_1,Buffer_2,Buffer_3,Buffer_4,Buffer_5,Buffer_6,Buffer_7,Buffer_8
  Constant : Constant  Value=0  OutDataTypeStr=uint8
  Equal : RelationalOperator  Operator===  OutDataTypeStr=boolean  RndMeth=Simplest
  Subsystem : Subsystem
  Terminator : Terminator
  msg_count>2_DEBUG : Subsystem
  CAN1_msg : Outport  OutDataTypeStr=Bus: msg_buffer_type
  Msg_Count_CAN1 : Outport  Port=2
  CAN1_msg_coherent : Outport  Port=3  OutputWhenDisabled=reset  InitialOutput=0
  wires:
  Subsystem/1(basic_cycle) -> Terminator/1
  Constant/1 -> Bus Creator/1
  Bus Creator/1 -> CAN1_msg/1
  Subsystem/2(msg_count) -> Msg_Count_CAN1/1, msg_count>2_DEBUG/1(msg_c)
  Bus Selector/1 -> Subsystem/1(Msg_Temporal_Data)  "<Buffer_1>"
  Subsystem/3(board_id) -> Equal/1
  Bus Selector/4 -> Bus Creator/4  "<Buffer_4>"
  Bus Selector/8 -> Bus Creator/8  "<Buffer_8>"
  Bus Selector/7 -> Bus Creator/7  "<Buffer_7>"
  Bus Selector/5 -> Bus Creator/5  "<Buffer_5>"
  Bus Selector/6 -> Bus Creator/6  "<Buffer_6>"
  expected_board_id/1 -> Equal/2
  Equal/1 -> CAN1_msg_coherent/1
  CAN1_Rx_msg/1 -> Bus Selector/1
  Bus Selector/3 -> Bus Creator/3  "<Buffer_3>"
  Bus Selector/2 -> Bus Creator/2  "<Buffer_2>"

== system HANcoder_E407_TTA_Group2/HANcoder STM32 Target - E407-STM32 algorithm/TTA CAN System/TTA System/Matrix Cycle Manager/Controller Matrix Cycle/controller basic cycle 0/COMP Task - Vote2 check/Process_Messages/Demux message CAN1 and check coherence1 ==
  CAN2_Rx_msg : Inport  OutDataTypeStr=Bus: msg_buffer_type
  expected_board_id : Inport  Port=2
  Enable : EnablePort
  Bus Creator : BusCreator  Inputs=8  OutDataTypeStr=Bus: msg_buffer_type
  Bus Selector : BusSelector  OutputSignals=Buffer_1,Buffer_2,Buffer_3,Buffer_4,Buffer_5,Buffer_6,Buffer_7,Buffer_8
  Constant : Constant  Value=0  OutDataTypeStr=uint8
  Equal : RelationalOperator  Operator===  OutDataTypeStr=boolean  RndMeth=Simplest
  Subsystem : Subsystem
  Terminator : Terminator
  msg_count>2_DEBUG : Subsystem
  CAN2_msg_coherent : Outport  OutputWhenDisabled=reset  InitialOutput=0
  Msg_Count_CAN2 : Outport  Port=2
  CAN2_msg : Outport  Port=3  OutDataTypeStr=Bus: msg_buffer_type
  wires:
  Subsystem/1(basic_cycle) -> Terminator/1
  Constant/1 -> Bus Creator/1
  Bus Creator/1 -> CAN2_msg/1
  Subsystem/2(msg_count) -> Msg_Count_CAN2/1, msg_count>2_DEBUG/1(msg_c)
  Bus Selector/1 -> Subsystem/1(Msg_Temporal_Data)  "<Buffer_1>"
  Subsystem/3(board_id) -> Equal/1
  Bus Selector/4 -> Bus Creator/4  "<Buffer_4>"
  Bus Selector/8 -> Bus Creator/8  "<Buffer_8>"
  Bus Selector/7 -> Bus Creator/7  "<Buffer_7>"
  Bus Selector/5 -> Bus Creator/5  "<Buffer_5>"
  Bus Selector/6 -> Bus Creator/6  "<Buffer_6>"
  expected_board_id/1 -> Equal/2
  Equal/1 -> CAN2_msg_coherent/1
  CAN2_Rx_msg/1 -> Bus Selector/1
  Bus Selector/3 -> Bus Creator/3  "<Buffer_3>"
  Bus Selector/2 -> Bus Creator/2  "<Buffer_2>"

== system HANcoder_E407_TTA_Group2/HANcoder STM32 Target - E407-STM32 algorithm/TTA CAN System/TTA System/Matrix Cycle Manager/Controller Matrix Cycle/controller basic cycle 0/COMP Task - Vote3 check/Process_Messages/Demux message CAN1 and check coherence ==
  CAN1_Rx_msg : Inport  OutDataTypeStr=Bus: msg_buffer_type
  expected_board_id : Inport  Port=2
  Enable : EnablePort
  Bus Creator : BusCreator  Inputs=8  OutDataTypeStr=Bus: msg_buffer_type
  Bus Selector : BusSelector  OutputSignals=Buffer_1,Buffer_2,Buffer_3,Buffer_4,Buffer_5,Buffer_6,Buffer_7,Buffer_8
  Constant : Constant  Value=0  OutDataTypeStr=uint8
  Equal : RelationalOperator  Operator===  OutDataTypeStr=boolean  RndMeth=Simplest
  Subsystem : Subsystem
  Terminator : Terminator
  msg_count>2_DEBUG : Subsystem
  CAN1_msg : Outport  OutDataTypeStr=Bus: msg_buffer_type
  Msg_Count_CAN1 : Outport  Port=2
  CAN1_msg_coherent : Outport  Port=3  OutputWhenDisabled=reset  InitialOutput=0
  wires:
  Bus Selector/2 -> Bus Creator/2  "<Buffer_2>"
  Bus Selector/3 -> Bus Creator/3  "<Buffer_3>"
  CAN1_Rx_msg/1 -> Bus Selector/1
  Equal/1 -> CAN1_msg_coherent/1
  expected_board_id/1 -> Equal/2
  Bus Selector/6 -> Bus Creator/6  "<Buffer_6>"
  Bus Selector/5 -> Bus Creator/5  "<Buffer_5>"
  Bus Selector/7 -> Bus Creator/7  "<Buffer_7>"
  Bus Selector/8 -> Bus Creator/8  "<Buffer_8>"
  Bus Selector/4 -> Bus Creator/4  "<Buffer_4>"
  Subsystem/3(board_id) -> Equal/1
  Bus Selector/1 -> Subsystem/1(Msg_Temporal_Data)  "<Buffer_1>"
  Subsystem/2(msg_count) -> Msg_Count_CAN1/1, msg_count>2_DEBUG/1(msg_c)
  Bus Creator/1 -> CAN1_msg/1
  Constant/1 -> Bus Creator/1
  Subsystem/1(basic_cycle) -> Terminator/1

== system HANcoder_E407_TTA_Group2/HANcoder STM32 Target - E407-STM32 algorithm/TTA CAN System/TTA System/Matrix Cycle Manager/Controller Matrix Cycle/controller basic cycle 0/COMP Task - Vote3 check/Process_Messages/Demux message CAN1 and check coherence1 ==
  CAN2_Rx_msg : Inport  OutDataTypeStr=Bus: msg_buffer_type
  expected_board_id : Inport  Port=2
  Enable : EnablePort
  Bus Creator : BusCreator  Inputs=8  OutDataTypeStr=Bus: msg_buffer_type
  Bus Selector : BusSelector  OutputSignals=Buffer_1,Buffer_2,Buffer_3,Buffer_4,Buffer_5,Buffer_6,Buffer_7,Buffer_8
  Constant : Constant  Value=0  OutDataTypeStr=uint8
  Equal : RelationalOperator  Operator===  OutDataTypeStr=boolean  RndMeth=Simplest
  Subsystem : Subsystem
  Terminator : Terminator
  msg_count>2_DEBUG : Subsystem
  CAN2_msg_coherent : Outport  OutputWhenDisabled=reset  InitialOutput=0
  Msg_Count_CAN2 : Outport  Port=2
  CAN2_msg : Outport  Port=3  OutDataTypeStr=Bus: msg_buffer_type
  wires:
  Bus Selector/2 -> Bus Creator/2  "<Buffer_2>"
  Bus Selector/3 -> Bus Creator/3  "<Buffer_3>"
  CAN2_Rx_msg/1 -> Bus Selector/1
  Equal/1 -> CAN2_msg_coherent/1
  expected_board_id/1 -> Equal/2
  Bus Selector/6 -> Bus Creator/6  "<Buffer_6>"
  Bus Selector/5 -> Bus Creator/5  "<Buffer_5>"
  Bus Selector/7 -> Bus Creator/7  "<Buffer_7>"
  Bus Selector/8 -> Bus Creator/8  "<Buffer_8>"
  Bus Selector/4 -> Bus Creator/4  "<Buffer_4>"
  Subsystem/3(board_id) -> Equal/1
  Bus Selector/1 -> Subsystem/1(Msg_Temporal_Data)  "<Buffer_1>"
  Subsystem/2(msg_count) -> Msg_Count_CAN2/1, msg_count>2_DEBUG/1(msg_c)
  Bus Creator/1 -> CAN2_msg/1
  Constant/1 -> Bus Creator/1
  Subsystem/1(basic_cycle) -> Terminator/1

== system HANcoder_E407_TTA_Group2/HANcoder STM32 Target - E407-STM32 algorithm/TTA CAN System/TTA System/Matrix Cycle Manager/Controller Matrix Cycle/controller basic cycle 0/COMP Task - Vote4 check/Process_Messages/Demux message CAN1 and check coherence ==
  CAN1_Rx_msg : Inport  OutDataTypeStr=Bus: msg_buffer_type
  expected_board_id : Inport  Port=2
  Enable : EnablePort
  Bus Creator : BusCreator  Inputs=8  OutDataTypeStr=Bus: msg_buffer_type
  Bus Selector : BusSelector  OutputSignals=Buffer_1,Buffer_2,Buffer_3,Buffer_4,Buffer_5,Buffer_6,Buffer_7,Buffer_8
  Constant : Constant  Value=0  OutDataTypeStr=uint8
  Equal : RelationalOperator  Operator===  OutDataTypeStr=boolean  RndMeth=Simplest
  Subsystem : Subsystem
  Terminator : Terminator
  msg_count>2_DEBUG : Subsystem
  CAN1_msg : Outport  OutDataTypeStr=Bus: msg_buffer_type
  Msg_Count_CAN1 : Outport  Port=2
  CAN1_msg_coherent : Outport  Port=3  OutputWhenDisabled=reset  InitialOutput=0
  wires:
  Bus Selector/2 -> Bus Creator/2  "<Buffer_2>"
  Bus Selector/3 -> Bus Creator/3  "<Buffer_3>"
  CAN1_Rx_msg/1 -> Bus Selector/1
  Equal/1 -> CAN1_msg_coherent/1
  expected_board_id/1 -> Equal/2
  Bus Selector/6 -> Bus Creator/6  "<Buffer_6>"
  Bus Selector/5 -> Bus Creator/5  "<Buffer_5>"
  Bus Selector/7 -> Bus Creator/7  "<Buffer_7>"
  Bus Selector/8 -> Bus Creator/8  "<Buffer_8>"
  Bus Selector/4 -> Bus Creator/4  "<Buffer_4>"
  Subsystem/3(board_id) -> Equal/1
  Bus Selector/1 -> Subsystem/1(Msg_Temporal_Data)  "<Buffer_1>"
  Subsystem/2(msg_count) -> Msg_Count_CAN1/1, msg_count>2_DEBUG/1(msg_c)
  Bus Creator/1 -> CAN1_msg/1
  Constant/1 -> Bus Creator/1
  Subsystem/1(basic_cycle) -> Terminator/1
